simulink model "WorkshopB_1_Code_14"  (Simulink 8.3)
settings: Solver=ode45  SolverMode=SingleTasking  StartTime=0.0  StopTime=2  RelTol=1e-3
undefined symbols (not defined in the file): DiscIntNeverNeededParam, dm, Dpos, Fc, Ipos, Jeq, Kemf, Km, Max_Speed, n, Npos, Ppos, R, sigbuilder_block, Ts
settings Model: Creator=sofianh  LastModifiedBy=diegogm  CovModelRefEnable=off
settings DataIOCC: SignalLoggingSaveFormat=Dataset
settings OptimizationCC: BlockReduction=off  BooleanDataType=off
settings DebuggingCC: SaveWithParameterizedLinksMsg=none  SignalResolutionControl=TryResolveAllWithWarning  SolverPrmCheckMsg=none  FrameProcessingCompatibilityMsg=error  StateNameClashWarn=none
settings HardwareCC: TargetUnknown=on
settings GRTTargetCC: CombineOutputUpdateFcns=on  GRTInterface=off

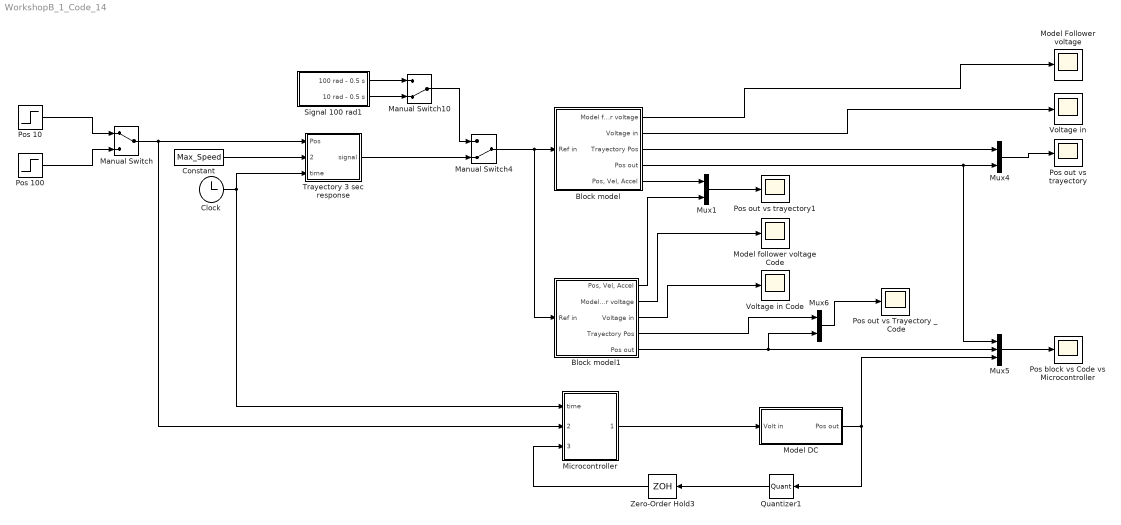
== system WorkshopB_1_Code_14 ==
  Block model : Subsystem
  Block model1 : Subsystem
  Clock : Clock
  Constant : Constant  Value=Max_Speed
  Manual Switch : ManualSwitch
  Manual Switch10 : ManualSwitch  CurrentSetting=0
  Manual Switch4 : ManualSwitch  CurrentSetting=0
  Microcontroller : MATLAB Function  TreatAsAtomicUnit=on  SystemSampleTime=Ts
      settings: PermitHierarchicalResolution=ParametersOnly
  "Model DC  " : Subsystem
  Model Follower voltage : Scope
      settings: TimeRange=auto  LimitDataPoints=on  MaxDataPoints=5000  SaveToWorkspace=off  SaveName=ScopeData2  YMin=-74.05416  YMax=524.30498  SampleTime=-1  DataFormat=Array
  Model follower voltage Code : Scope
      settings: TimeRange=auto  LimitDataPoints=on  MaxDataPoints=5000  SaveToWorkspace=off  SaveName=ScopeData3  YMin=-10  YMax=10  SampleTime=-1  DataFormat=Array
  Mux1 : Mux  Inputs=2
  Mux4 : Mux  Inputs=2
  Mux5 : Mux  Inputs=3
  Mux6 : Mux  Inputs=2
  Pos 10 : Step  Time=0  After=10  SampleTime=0
  Pos 100 : Step  Time=0  After=100  SampleTime=0
  "Pos block vs Code vs Microcontroller  " : Scope
      settings: TimeRange=auto  MaxDataPoints=5000  SaveToWorkspace=off  YMin=-1.25023  YMax=11.25205  SampleTime=-1
  "Pos out vs Trayectory _ Code " : Scope
      settings: TimeRange=auto  MaxDataPoints=5000  SaveToWorkspace=off  SaveName=ScopeData2  YMin=-1.25023  YMax=11.25205  SampleTime=-1
  Pos out vs trayectory : Scope
      settings: TimeRange=4  LimitDataPoints=on  MaxDataPoints=5000  SaveToWorkspace=off  SaveName=ScopeData3  YMin=-1.25022  YMax=11.252  SampleTime=-1  DataFormat=Array
  Pos out vs trayectory1 : Scope
      settings: TimeRange=4  LimitDataPoints=on  MaxDataPoints=5000  SaveToWorkspace=off  SaveName=ScopeData5  YMin=-12.50024  YMax=112.50212  SampleTime=-1  DataFormat=Array
  Quantizer1 : Quantizer  QuantizationInterval=Pulses  SampleTime=Ts
  Signal 100 rad1 : Subsystem  Tag=STV Subsys  LoadFcn=sigbuilder_block('load');  StartFcn=sigbuilder_block('start');  StopFcn=sigbuilder_block('stop');  ClipboardFcn=sigbuilder_block('clipboard');  mask(Sigbuilder block){}
      mask help: Simulink:masks:SigbuilderBlock_MD
      mask init:
      | if ~strcmp(get_param(bdroot(gcbh),'SimulationStatus'),'stopped') tuvar = sigbuilder_block('maskInit'); end
      settings: CopyFcn=sigbuilder_block('copy');  DeleteFcn=sigbuilder_block('delete');  ModelCloseFcn=sigbuilder_block('modelClose');  PreSaveFcn=sigbuilder_block('preSave');  PauseFcn=sigbuilder_block('pause');  ContinueFcn=sigbuilder_block('continue');  NameChangeFcn=sigbuilder_block('namechange');  OpenFcn=sigbuilder_block('open',[437.6 199.2 550.4 400 ]);  CloseFcn=sigbuilder_block('close');
      mask Display: plot(0, 0, 100, 100,[2, 2, 32, 32, 2], [68, 8, 8, 68, 68],[32, 2], [38, 38], [32, 19, 2],[53, 60, 44], [32, 17, 17, 2],[16, 16, 31, 31]);txt = getActiveGroup(gcbh);text(2, 100, txt,'verticalAlignment', 'top');
  Trayectory 3 sec response : MATLAB Function  TreatAsAtomicUnit=on  SystemSampleTime=1e-3
      settings: PermitHierarchicalResolution=ParametersOnly
  Voltage in : Scope
      settings: TimeRange=auto  LimitDataPoints=on  MaxDataPoints=5000  SaveToWorkspace=off  SaveName=ScopeData4  YMin=-10.38658  YMax=11.94268  SampleTime=-1  DataFormat=Array
  "Voltage in Code " : Scope
      settings: TimeRange=auto  LimitDataPoints=on  MaxDataPoints=5000  SaveToWorkspace=off  SaveName=ScopeData4  YMin=-10  YMax=10  SampleTime=-1  DataFormat=Array
  Zero-Order Hold3 : ZeroOrderHold  SampleTime=Ts
  wires:
  Clock/1 -> Microcontroller/1(time), Trayectory 3 sec response/3(time)
  Pos 10/1 -> Manual Switch/1
  Pos 100/1 -> Manual Switch/2
  Manual Switch/1 -> Microcontroller/2(Pos_aim), Trayectory 3 sec response/1(Pos)
  Block model/1(Model follower voltage) -> Model Follower voltage/1
  Mux4/1 -> Pos out vs trayectory/1
  Trayectory 3 sec response/1(signal) -> Manual Switch4/2
  Constant/1 -> Trayectory 3 sec response/2(Speed_ref)
  Signal 100 rad1/1(100 rad - 0.5 s) -> Manual Switch10/1
  Signal 100 rad1/2(10 rad - 0.5 s) -> Manual Switch10/2
  Manual Switch10/1 -> Manual Switch4/1
  Manual Switch4/1 -> Block model1/1(Ref in), Block model/1(Ref in)
  Mux5/1 -> "Pos block vs Code vs Microcontroller  "/1
  Mux6/1 -> "Pos out vs Trayectory _ Code "/1
  Block model/2(Voltage in) -> Voltage in/1
  Block model/3(Trayectory Pos) -> Mux4/1
  Block model/4("Pos out ") -> Mux5/1, Mux4/2
  Block model1/5("Pos out ") -> Mux6/2, Mux5/2
  Block model1/4(Trayectory Pos) -> Mux6/1
  Block model1/2(Model follower voltage) -> Model follower voltage Code/1
  Block model1/3(Voltage in) -> "Voltage in Code "/1
  "Model DC  "/1(Pos out) -> Mux5/3, Quantizer1/1
  Quantizer1/1 -> Zero-Order Hold3/1
  Microcontroller/1(Voltage) -> "Model DC  "/1("Volt in ")
  Zero-Order Hold3/1 -> Microcontroller/3(Output)
  Mux1/1 -> Pos out vs trayectory1/1
  Block model1/1("Pos, Vel, Accel ") -> Mux1/2
  Block model/5("Pos, Vel, Accel ") -> Mux1/1

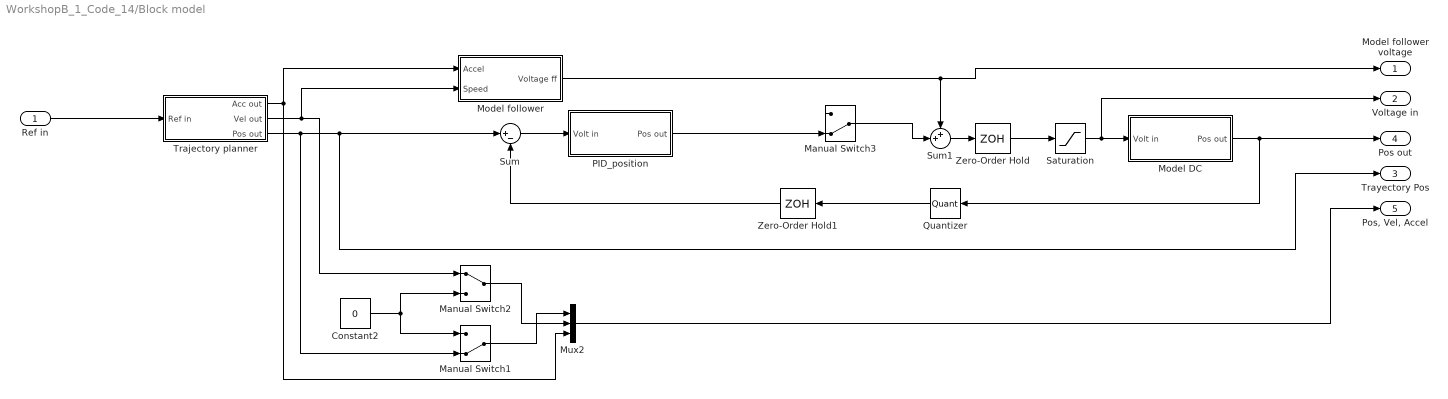
== system WorkshopB_1_Code_14/Block model ==
  Ref in : Inport
  Constant2 : Constant  Value=0
  Manual Switch1 : ManualSwitch  CurrentSetting=0
  Manual Switch2 : ManualSwitch
  Manual Switch3 : ManualSwitch  CurrentSetting=0
  "Model DC " : Subsystem
  Model follower : Subsystem
  Mux2 : Mux  Inputs=3
  PID_position : Subsystem
  Quantizer : Quantizer  QuantizationInterval=Pulses  SampleTime=Ts
  Saturation : Saturate  UpperLimit=24  LowerLimit=-24
  Sum : Sum  Inputs=|+-
  Sum1 : Sum  Inputs=++|
  Trajectory planner : Subsystem
  Zero-Order Hold : ZeroOrderHold  SampleTime=Ts
  Zero-Order Hold1 : ZeroOrderHold  SampleTime=Ts
  Model follower voltage : Outport
  Voltage in : Outport  Port=2
  Trayectory Pos : Outport  Port=3
  "Pos out " : Outport  Port=4
  "Pos, Vel, Accel " : Outport  Port=5
  wires:
  Mux2/1 -> "Pos, Vel, Accel "/1
  Manual Switch1/1 -> Mux2/1
  Manual Switch2/1 -> Mux2/2
  Constant2/1 -> Manual Switch2/2, Manual Switch1/1
  Sum/1 -> PID_position/1(Volt in)
  "Model DC "/1(Pos out) -> "Pos out "/1, Quantizer/1
  Sum1/1 -> Zero-Order Hold/1
  Quantizer/1 -> Zero-Order Hold1/1
  Zero-Order Hold1/1 -> Sum/2
  Ref in/1 -> Trajectory planner/1(Ref in)
  Trajectory planner/3("Pos out ") -> Trayectory Pos/1, Sum/1, Manual Switch1/2
  Trajectory planner/2(Vel out) -> Manual Switch2/1, Model follower/2(Speed)
  Trajectory planner/1("Acc out ") -> Model follower/1(Accel), Mux2/3
  Model follower/1(Voltage ff) -> Model follower voltage/1, Sum1/1
  PID_position/1(Pos out) -> Manual Switch3/2
  Manual Switch3/1 -> Sum1/2
  Zero-Order Hold/1 -> Saturation/1
  Saturation/1 -> Voltage in/1, "Model DC "/1("Volt in ")

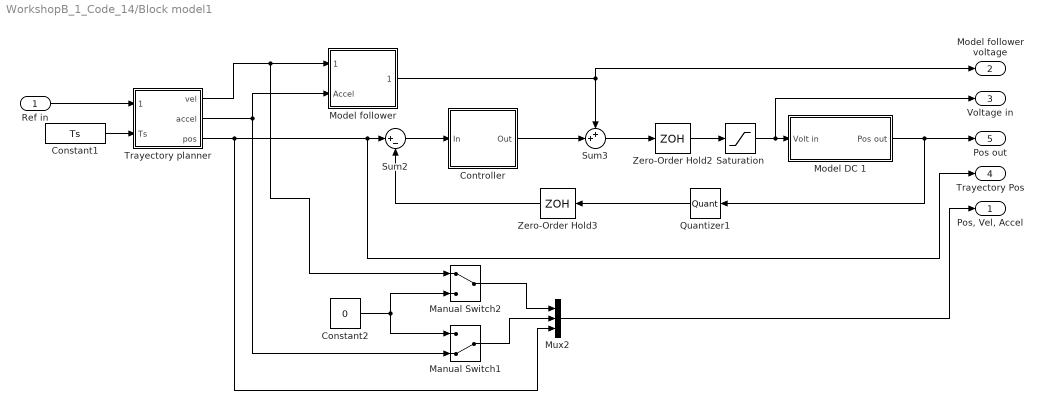
== system WorkshopB_1_Code_14/Block model1 ==
  Ref in : Inport
  Constant1 : Constant  Value=Ts
  Constant2 : Constant  Value=0
  "Controller " : MATLAB Function  TreatAsAtomicUnit=on  SystemSampleTime=Ts
      settings: PermitHierarchicalResolution=ParametersOnly
  Manual Switch1 : ManualSwitch  CurrentSetting=0
  Manual Switch2 : ManualSwitch
  Model DC 1 : Subsystem
  "Model follower " : MATLAB Function  TreatAsAtomicUnit=on  SystemSampleTime=Ts
      settings: PermitHierarchicalResolution=ParametersOnly
  Mux2 : Mux  Inputs=3
  Quantizer1 : Quantizer  QuantizationInterval=Pulses  SampleTime=Ts
  Saturation : Saturate  UpperLimit=24  LowerLimit=-24
  Sum2 : Sum  Inputs=|+-
  Sum3 : Sum  Inputs=++|
  Trayectory planner : MATLAB Function  TreatAsAtomicUnit=on  SystemSampleTime=Ts
      settings: PermitHierarchicalResolution=ParametersOnly
  Zero-Order Hold2 : ZeroOrderHold  SampleTime=Ts
  Zero-Order Hold3 : ZeroOrderHold  SampleTime=Ts
  "Pos, Vel, Accel " : Outport
  Model follower voltage : Outport  Port=2
  Voltage in : Outport  Port=3
  Trayectory Pos : Outport  Port=4
  "Pos out " : Outport  Port=5
  wires:
  Ref in/1 -> Trayectory planner/1(signal_in)
  Constant1/1 -> Trayectory planner/2(Ts)
  Sum2/1 -> "Controller "/1(In)
  Model DC 1/1(Pos out) -> "Pos out "/1, Quantizer1/1
  Sum3/1 -> Zero-Order Hold2/1
  Quantizer1/1 -> Zero-Order Hold3/1
  Zero-Order Hold3/1 -> Sum2/2
  "Model follower "/1(Voltage) -> Model follower voltage/1, Sum3/1
  "Controller "/1(Out) -> Sum3/2
  Mux2/1 -> "Pos, Vel, Accel "/1
  Constant2/1 -> Manual Switch2/2, Manual Switch1/1
  Trayectory planner/2(accel) -> "Model follower "/2(Accel), Manual Switch1/2
  Trayectory planner/1(vel) -> Manual Switch2/1, "Model follower "/1(Speed)
  Trayectory planner/3(pos) -> Trayectory Pos/1, Sum2/1, Mux2/3
  Manual Switch2/1 -> Mux2/1
  Manual Switch1/1 -> Mux2/2
  Zero-Order Hold2/1 -> Saturation/1
  Saturation/1 -> Voltage in/1, Model DC 1/1("Volt in ")

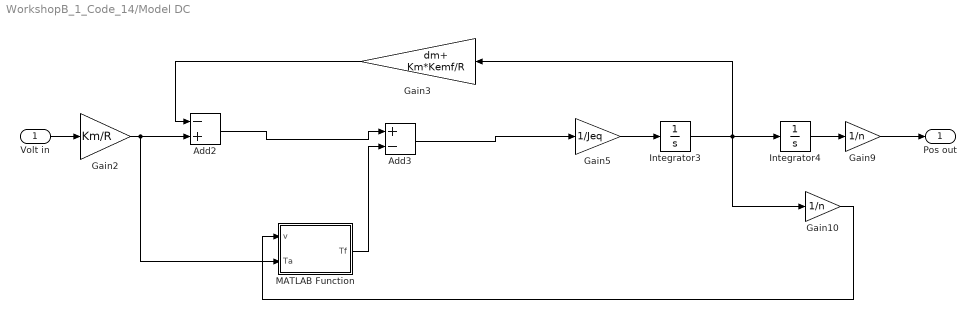
== system WorkshopB_1_Code_14/Model DC   ==
  "Volt in " : Inport
  Add2 : Sum  Inputs=-+
  Add3 : Sum  Inputs=+-
  Gain10 : Gain  Gain=1/n
  Gain2 : Gain  Gain=Km/R
  Gain3 : Gain  Gain=dm+ Km*Kemf/R
  Gain5 : Gain  Gain=1/Jeq
  Gain9 : Gain  Gain=1/n
  Integrator3 : Integrator
  Integrator4 : Integrator
  MATLAB Function : MATLAB Function  TreatAsAtomicUnit=on
      settings: PermitHierarchicalResolution=ParametersOnly
  Pos out : Outport
  wires:
  Gain2/1 -> MATLAB Function/2(Ta), Add2/2
  Integrator3/1 -> Integrator4/1, Gain10/1, Gain3/1
  Gain3/1 -> Add2/1
  Gain5/1 -> Integrator3/1
  Integrator4/1 -> Gain9/1
  Gain10/1 -> MATLAB Function/1(v)
  Add3/1 -> Gain5/1
  Add2/1 -> Add3/1
  MATLAB Function/1(Tf) -> Add3/2
  "Volt in "/1 -> Gain2/1
  Gain9/1 -> Pos out/1

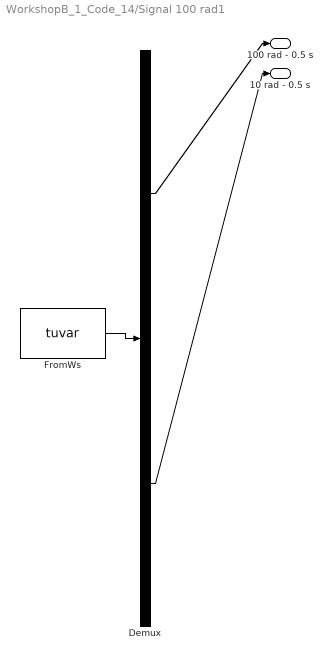
== system WorkshopB_1_Code_14/Signal 100 rad1 ==
  Demux : Demux  Tag=STV Demux  Outputs=2
  FromWs : FromWorkspace  Tag=STV FromWs  VariableName=tuvar  SampleTime=0  SigBuilderData=DataTag0  VnvData=DataTag1
      SigBuilderData=|
      | common.afterFinalStr = 'Extrapolate'
      | common.sampleTime = 0
      | dataSet.timeRange = [0 2]
      | dataSet.name = 'Group 1'
      | sbobj.Groups.Name = 'Group 1'
      | sbobj.Groups.Signals(1).Name = '100 rad - 0.5 s'
      | sbobj.Groups.Signals(1).XData = [0 0.5 0.5 1 1 1.5 1.5 2]
      | sbobj.Groups.Signals(1).YData = [200 200 0 0 -200 -200 0 0]
      | sbobj.Groups.Signals(2).Name = '10 rad - 0.5 s'
      | sbobj.Groups.Signals(2).XData = [0 0.5 0.5 1 1 1.5 1.5 2]
      | sbobj.Groups.Signals(2).YData = [20 20 0 0 -20 -20 0 0]
      | sbobj.Groups.TimeRange = [0 2]
  100 rad - 0.5 s : Outport  Tag=STV Outport
  10 rad - 0.5 s : Outport  Tag=STV Outport  Port=2
  wires:
  FromWs/1 -> Demux/1
  Demux/1 -> 100 rad - 0.5 s/1
  Demux/2 -> 10 rad - 0.5 s/1

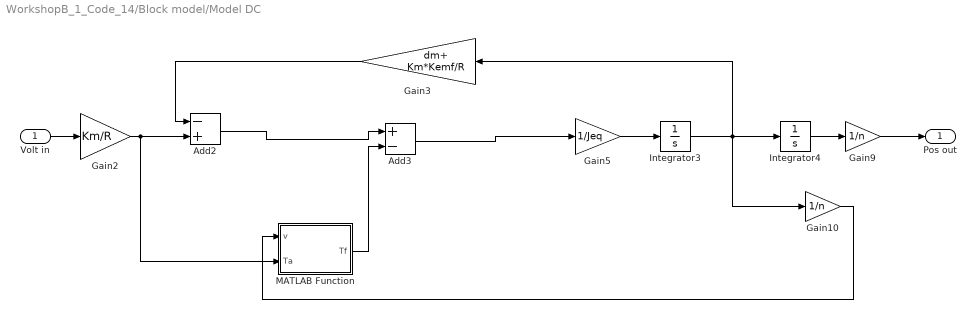
== system WorkshopB_1_Code_14/Block model/Model DC  ==
  "Volt in " : Inport
  Add2 : Sum  Inputs=-+
  Add3 : Sum  Inputs=+-
  Gain10 : Gain  Gain=1/n
  Gain2 : Gain  Gain=Km/R
  Gain3 : Gain  Gain=dm+ Km*Kemf/R
  Gain5 : Gain  Gain=1/Jeq
  Gain9 : Gain  Gain=1/n
  Integrator3 : Integrator
  Integrator4 : Integrator
  MATLAB Function : MATLAB Function  TreatAsAtomicUnit=on
      settings: PermitHierarchicalResolution=ParametersOnly
  Pos out : Outport
  wires:
  Gain2/1 -> MATLAB Function/2(Ta), Add2/2
  Integrator3/1 -> Integrator4/1, Gain10/1, Gain3/1
  Gain3/1 -> Add2/1
  Gain5/1 -> Integrator3/1
  Integrator4/1 -> Gain9/1
  Gain10/1 -> MATLAB Function/1(v)
  Add3/1 -> Gain5/1
  Add2/1 -> Add3/1
  MATLAB Function/1(Tf) -> Add3/2
  "Volt in "/1 -> Gain2/1
  Gain9/1 -> Pos out/1

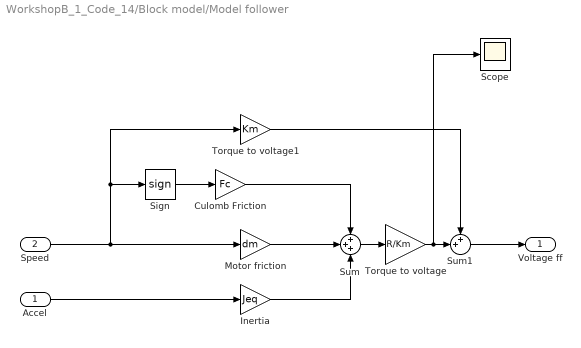
== system WorkshopB_1_Code_14/Block model/Model follower ==
  Accel : Inport
  Speed : Inport  Port=2
  Culomb Friction : Gain  Gain=Fc
  "Inertia " : Gain  Gain=Jeq
  Motor friction : Gain  Gain=dm
  Scope : Scope
      settings: TimeRange=auto  LimitDataPoints=on  MaxDataPoints=5000  SaveToWorkspace=off  SaveName=ScopeData5  YMin=-10  YMax=10  SampleTime=-1  DataFormat=Array
  Sign : Signum
  Sum : Sum  Inputs=+++
  Sum1 : Sum  Inputs=++|
  Torque to voltage : Gain  Gain=R/Km
  Torque to voltage1 : Gain  Gain=Km
  Voltage ff : Outport
  wires:
  Accel/1 -> "Inertia "/1
  Speed/1 -> Torque to voltage1/1, Sign/1, Motor friction/1
  "Inertia "/1 -> Sum/3
  Motor friction/1 -> Sum/2
  Sum/1 -> Torque to voltage/1
  Torque to voltage1/1 -> Sum1/1
  Torque to voltage/1 -> Scope/1, Sum1/2
  Sum1/1 -> Voltage ff/1
  Sign/1 -> Culomb Friction/1
  Culomb Friction/1 -> Sum/1

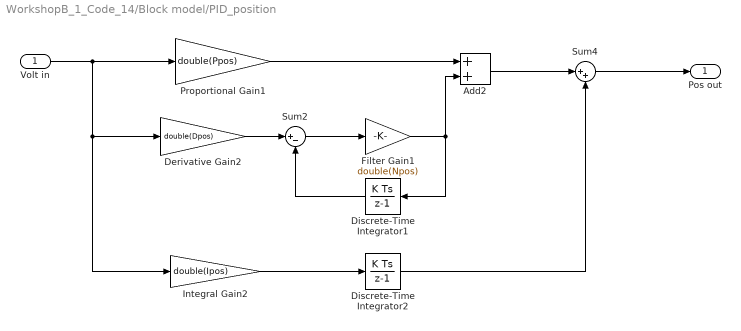
== system WorkshopB_1_Code_14/Block model/PID_position ==
  Volt in : Inport
  Add2 : Sum
  Derivative Gain2 : Gain  Gain=double(Dpos)
  Discrete-Time Integrator1 : DiscreteIntegrator  InitialConditionSetting=State (most efficient)  SampleTime=Ts  ICPrevOutput=DiscIntNeverNeededParam  ICPrevScaledInput=DiscIntNeverNeededParam
  Discrete-Time Integrator2 : DiscreteIntegrator  InitialConditionSetting=State (most efficient)  SampleTime=Ts  ICPrevOutput=DiscIntNeverNeededParam  ICPrevScaledInput=DiscIntNeverNeededParam
  Filter Gain1 : Gain  Gain=double(Npos)
  Integral Gain2 : Gain  Gain=double(Ipos)
  Proportional Gain1 : Gain  Gain=double(Ppos)
  Sum2 : Sum  Inputs=|+-
  Sum4 : Sum  Inputs=|++
  Pos out : Outport
  wires:
  Discrete-Time Integrator2/1 -> Sum4/2
  Add2/1 -> Sum4/1
  Volt in/1 -> Integral Gain2/1, Derivative Gain2/1, Proportional Gain1/1
  Discrete-Time Integrator1/1 -> Sum2/2
  Sum2/1 -> Filter Gain1/1
  Derivative Gain2/1 -> Sum2/1
  Proportional Gain1/1 -> Add2/1
  Filter Gain1/1 -> Discrete-Time Integrator1/1, Add2/2
  Integral Gain2/1 -> Discrete-Time Integrator2/1
  Sum4/1 -> Pos out/1

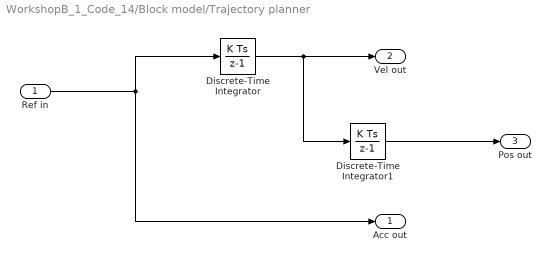
== system WorkshopB_1_Code_14/Block model/Trajectory planner ==
  Ref in : Inport
  Discrete-Time Integrator : DiscreteIntegrator  InitialConditionSetting=State (most efficient)  SampleTime=Ts  ICPrevOutput=DiscIntNeverNeededParam  ICPrevScaledInput=DiscIntNeverNeededParam
  Discrete-Time Integrator1 : DiscreteIntegrator  InitialConditionSetting=State (most efficient)  SampleTime=Ts  ICPrevOutput=DiscIntNeverNeededParam  ICPrevScaledInput=DiscIntNeverNeededParam
  "Acc out " : Outport
  Vel out : Outport  Port=2
  "Pos out " : Outport  Port=3
  wires:
  Discrete-Time Integrator/1 -> Discrete-Time Integrator1/1, Vel out/1
  Ref in/1 -> Discrete-Time Integrator/1, "Acc out "/1
  Discrete-Time Integrator1/1 -> "Pos out "/1

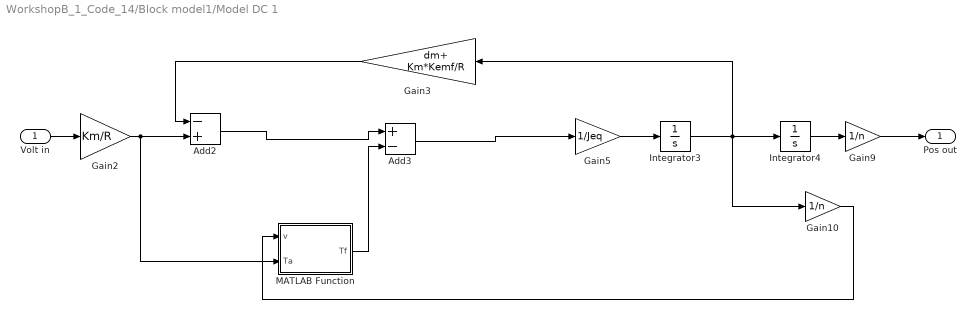
== system WorkshopB_1_Code_14/Block model1/Model DC 1 ==
  "Volt in " : Inport
  Add2 : Sum  Inputs=-+
  Add3 : Sum  Inputs=+-
  Gain10 : Gain  Gain=1/n
  Gain2 : Gain  Gain=Km/R
  Gain3 : Gain  Gain=dm+ Km*Kemf/R
  Gain5 : Gain  Gain=1/Jeq
  Gain9 : Gain  Gain=1/n
  Integrator3 : Integrator
  Integrator4 : Integrator
  MATLAB Function : MATLAB Function  TreatAsAtomicUnit=on
      settings: PermitHierarchicalResolution=ParametersOnly
  Pos out : Outport
  wires:
  Gain2/1 -> MATLAB Function/2(Ta), Add2/2
  Integrator3/1 -> Integrator4/1, Gain10/1, Gain3/1
  Gain3/1 -> Add2/1
  Gain5/1 -> Integrator3/1
  Integrator4/1 -> Gain9/1
  Gain10/1 -> MATLAB Function/1(v)
  Add3/1 -> Gain5/1
  Add2/1 -> Add3/1
  MATLAB Function/1(Tf) -> Add3/2
  "Volt in "/1 -> Gain2/1
  Gain9/1 -> Pos out/1

== matlab function Microcontroller ==
  data: time input double; Pos_aim input double; Output input double; Voltage output double
function Voltage   = Planner(time, Pos_aim,Output)
    
    %%%%%%%%%%%%%%%%%%%%%%%%%
    %%Parameter declaration%%
    %%%%%%%%%%%%%%%%%%%%%%%%%

    R = 112;
    Km = 69.7E-3;
    Kemf = 1/(137*2*pi/60);
    dm = 3.8E-6;
    Jm = 7.46/(1000*100^2);
    J1 = 1.8E-5;
    J2 = 1.8E-5;
    n = 1;
    Jeq = Jm + (J1+J2)/(n^2);
    %Calculated parameters for the DC motor used in the workshops
    eps_Jeq = 0.6; % Scaling factor for inertia
    eps_dm = 3.56; % scaling blabals
    
    Jeq = eps_Jeq*Jeq;
    dm = dm*eps_dm; 
    %Coulomb friction
    Fc = 0.0013;
    
    %Sampling time
    Ts = 5e-3;
    %%%%%%%%%%%%%%%%%%%%%%%%%%%%%%%%%%%%%%%%%%
    %%Trayectory planner - Signal generation%%
    %%%%%%%%%%%%%%%%%%%%%%%%%%%%%%%%%%%%%%%%%%
    
    %Define a rising time. The motor will be accelerating during 0.5 s.
    %Then it will have 0 acceleration over 0.5 s. Last step would be that
    %it accelerate in the opposite direction for 0.5 s. This acceleration
    %will be one such that it will never pass the maximum acceleration
    %(calculated in the following lines) and that ensures that the final
    %position is the one desired. 
    
    %Motor characteristics - from datasheet. We use a margin of 20% as the
    %PID controller will need some margins for operate correctly. 
    MaxCurrent = 0.182*0.8;
    MaxVoltage = 24*0.8;
    
    %Max dynamics
    Max_Speed_ref = MaxVoltage/Kemf;
    Max_Accel_ref = Km*MaxCurrent/Jeq;
    
    %Definition of trising
    trising = 0.5;
    
    %We calculate the speed and acceleration that we need to get to the
    %position given the trising time. 
    Max_Speed = Pos_aim/(2*trising);
    Max_Accel = Max_Speed/trising;
    
    %Check that we are inside the Max_acceleration and Max_speed boundaries
    if Max_Speed > Max_Speed_ref || Max_Accel > Max_Accel_ref
        disp('Error, Speed/Accel too high')
        pause();
    end 
    
    %Definition of the time that the motor will have 0 acceleration
    t_est = (Pos_aim - Max_Speed*trising)/Max_Speed;
    
    %If we haven't reached the trising time, the motor accelerates
    if time < trising
        signal_accel = Max_Accel;
    %If we reach this values, and have not reached t_est time, the motor
    %has 0 acceleration
    elseif time >= trising && time < (trising + t_est)
        signal_accel = 0; 
    %If we pass t_est, then it accelerates again but inversely
    elseif time >= (trising + t_est) && time < (2*trising + t_est)
        signal_accel = - Max_Accel;
    %when it has accelerated during trising, the acceleration remains
    %steady in 0.
    else
        signal_accel = 0;
    end
    
    %%%%%%%%%%%%%%%%%%%%%%%%%%%%%%%%%%%%%%%%%%%%%%%%%
    %%Trayectory planner - Acceleration integration%%
    %%%%%%%%%%%%%%%%%%%%%%%%%%%%%%%%%%%%%%%%%%%%%%%%%
    
    %We need to integrate the acceleration: once to get the velocity and
    %twice to get the position. This is done, in the discrete time: 
    %
    %   - Speed = (Ts/(z-1))*Accel
    %   - Pos = (Ts/(z-1))*Speed
    %
    %Translated this to code-style language, we have: 
    %
    %   - Speed(n) = Ts*Accel(n) + Speed(n-1)
    %   - Pos(n) = Ts*Speed(n) + Pos(n-1)
    
    %We need to store values from previous calls of this function, then: 
    %Declaration of Speed(n_1)
    persistent outspeed_n_1;
    %Declaration of Pos(n_1)
    persistent outpos_n_1;
    
    %Initialization to 0 of these variables
    if isempty(outspeed_n_1)
        outspeed_n_1 = 0;
    end
    if isempty(outpos_n_1)
        outpos_n_1 = 0;
    end
    
    %The acceleration is not changed, we just need it to calculate the
    %Speed and the postion.
    Speed = signal_accel*Ts + outspeed_n_1;
    outspeed_n_1 = Speed;
    Position = Speed*Ts + outpos_n_1;
    outpos_n_1 = Position;
    
    %%%%%%%%%%%%%%%%%%%%%%%%%%%%%%%%%
    %%Model planner - inverse model%%
    %%%%%%%%%%%%%%%%%%%%%%%%%%%%%%%%%
    
    % We inverse the motor model to get the voltage we need to get a
    % certain acceleration and voltage.  
    Voltage_Planner = (Speed*dm + signal_accel*Jeq + sign(Speed)*Fc)*R/Km + Km*Speed; 
    
    %%%%%%%%%%%%%%%%%%%%
    %%PID - controller%%
    %%%%%%%%%%%%%%%%%%%%
    %
    %We calculated a PID controller for the DC motor model using Pole
    %Placement, implemented as a matlab function for both workshops A and
    %B. We did not need a fast-response controller. The controller we
    %designed is: 
    %
    %         758.5 z^2 - 1393 z + 640.5
    %   PID = ---------------------------
    %          z^2 - 0.9268 z - 0.07323
    %
    %Rewriting this in a code-style, we get: 
    %
    %Out(n) = In(n)*758.5 + In(n-1)*(-1393) + In(n-2)*640.5 - Out(n-1)*(-0.9268) - Out(n-2)*(-0.07323);
    
    %We need again to declare some variables as persistent, as they have to
    %be used in different iterations of the function
    persistent Out_n_1;
    persistent Out_n_2;
    persistent In_n_1;
    persistent In_n_2;
    
    %Initialization of persistent variables
    if isempty(Out_n_1)
        Out_n_1 = 0;
    end
    if isempty(Out_n_2)
        Out_n_2 = 0;
    end
    if isempty(In_n_1)
        In_n_1 = 0;
    end
    if isempty(In_n_2)
        In_n_2 = 0;
    end
    
    %Declaration of the parameters of the PID
    PID_den = [1 -0.9268 -0.07323];
    PID_num = [758.5 -1393 640.5];
    
    %Is an error PID so we need to substract the actual position from the
    %aimed position. 
    Error = Position - Output; 
    
    %Main PID function
    Voltage_Controller = Error*PID_num(1) + In_n_1*PID_num(2) + In_n_2*PID_num(3) - Out_n_1*PID_den(2) - Out_n_2*PID_den(3);
    
    %Store the values for next iterations
    In_n_2 = In_n_1;
    In_n_1 = Error;
    Out_n_2 = Out_n_1;
    Out_n_1 = Voltage_Controller;
    
    %The last step will be to add both voltages, from the controller and
    %the trayectory planner
    Voltage = Voltage_Controller + Voltage_Planner;
end

== matlab function Block model/Model DC /MATLAB Function ==
  data: v input double; Tf output double; Ta input double
function Tf = fcn(v,Ta)
Tc = 1e-3;
dv = 1e-1;
if abs(v) < dv
    if abs(Ta) > Tc
        Tf = Tc*sign(Ta);
    else
        Tf = Ta;
    end
else
    Tf = Tc*sign(v);
end

== matlab function Block model1/Controller  ==
  data: In input double; Out output double
function Out  = Planner(In)
    persistent Out_n_1;
    persistent Out_n_2;
    persistent In_n_1;
    persistent In_n_2;

    if isempty(Out_n_1)
        Out_n_1 = 0;
    end
    if isempty(Out_n_2)
        Out_n_2 = 0;
    end
    if isempty(In_n_1)
        In_n_1 = 0;
    end
    if isempty(In_n_2)
        In_n_2 = 0;
    end
    
    PID_den = [1 -0.9268 -0.07323];
    PID_num = [758.5 -1393 640.5];
    
    Out = In*PID_num(1) + In_n_1*PID_num(2) + In_n_2*PID_num(3) - Out_n_1*PID_den(2) - Out_n_2*PID_den(3);
    
    In_n_2 = In_n_1;
    In_n_1 = In;
    Out_n_2 = Out_n_1;
    Out_n_1 = Out;
    
end

== matlab function Trayectory 3 sec response ==
  data: Pos input double; Speed_ref input double; time input double; signal output double
function signal = Planner(Pos, Speed_ref, time)
    trising = 0.5;
    Max_Speed = Pos/(2*trising);
    Max_Accel = Max_Speed/trising;
    t_est = (Pos - Max_Speed*trising)/Max_Speed;
    if time < trising
        signal = Max_Accel;
    elseif time >= trising && time < (trising + t_est)
        signal = 0; 
    elseif time >= (trising + t_est) && time < (2*trising + t_est)
        signal = - Max_Accel;
    else
        signal = 0;
    end
end

== matlab function Model DC /MATLAB Function ==
  data: v input double; Tf output double; Ta input double
function Tf = fcn(v,Ta)
Tc = 1e-3;
dv = 1e-1;
if abs(v) < dv
    if abs(Ta) > Tc
        Tf = Tc*sign(Ta);
    else
        Tf = Ta;
    end
else
    Tf = Tc*sign(v);
end

== matlab function Block model1/Model DC 1/MATLAB Function ==
  data: v input double; Tf output double; Ta input double
function Tf = fcn(v,Ta)
Tc = 1e-3;
dv = 1e-1;
if abs(v) < dv
    if abs(Ta) > Tc
        Tf = Tc*sign(Ta);
    else
        Tf = Ta;
    end
else
    Tf = Tc*sign(v);
end

== matlab function Block model1/Model follower  ==
  data: Speed input double; Voltage output double; Accel input double
function Voltage  = Planner(Speed, Accel)

R = 112;
Km = 69.7E-3;
dm = 3.8E-6;
Jm = 7.46/(1000*100^2);
J1 = 1.8E-5;
J2 = 1.8E-5;
n = 1;
Jeq = Jm + (J1+J2)/(n^2);

eps_Jeq = 0.6; % Scaling factor for inertia
eps_dm = 3.56; % scaling blabals

Jeq = eps_Jeq*Jeq;
dm = dm*eps_dm; 

Fc = 0.0013;

Voltage = (Speed*dm + Accel*Jeq + sign(Speed)*Fc)*R/Km + Km*Speed; 
end

== matlab function Block model1/Trayectory planner ==
  data: vel output double; accel output double; signal_in input double; pos output double; Ts input double
function [ vel, accel, pos] = Planner(signal_in,Ts)
    
    persistent outvel_n_1;
    persistent outpos_n_1;

    if isempty(outvel_n_1)
        outvel_n_1 = 0;
    end
    if isempty(outpos_n_1)
        outpos_n_1 = 0;
    end
    accel = signal_in;
    vel = accel*Ts + outvel_n_1;
    outvel_n_1 = vel;
    pos = vel*Ts + outpos_n_1;
    outpos_n_1 = pos;
end
